simulink model "VMC_Integration"  (R2024a)
settings: Solver=FixedStepDiscrete  StartTime=0.0  StopTime=10.0  FixedStep=0.005  RelTol=1e-3
undefined symbols (not defined in the file): Degree_To_Rad_Factor
libraries: simulink x24, slpidlib x5
(part 3 of 3)

== system VMC_Integration/Traction_Control/LimitedSlipDifferential/Subsystem ==
  LSD_Enable : Inport
  Controller_Setting : Inport  Port=2
  Bus Selector : BusSelector  OutputSignals=TC_Controller.TC_PID.TC_P,TC_Controller.TC_PID.TC_I,TC_Controller.TC_PID.TC_D
  Constant15 : Constant  Value=100  OutDataTypeStr=single  SampleTime=-1
  Data Type Conversion : DataTypeConversion  OutDataTypeStr=single  SaturateOnIntegerOverflow=off  RndMeth=Floor
  Demux : Demux
  Logical Operator1 : Logic  Operator=NAND  AllPortsSameDT=off  OutDataTypeStr=boolean
  Logical Operator2 : Logic  Operator=NAND  AllPortsSameDT=off  OutDataTypeStr=boolean
  Mux5 : Mux  Inputs=5
  Terminator : Terminator
  PID_Setting : Outport
  wires:
  Demux/4 -> Logical Operator1/2
  Demux/2 -> Logical Operator2/1
  Bus Selector/2 -> Mux5/2  "<TC_I>"
  Data Type Conversion/1 -> Mux5/5
  Mux5/1 -> PID_Setting/1  "PID_ParaFL"
  Constant15/1 -> Mux5/4  "N"
  Logical Operator1/1 -> Data Type Conversion/1
  Demux/3 -> Logical Operator2/2
  Demux/1 -> Logical Operator1/1
  Bus Selector/3 -> Mux5/3  "<TC_D>"
  LSD_Enable/1 -> Demux/1
  Bus Selector/1 -> Mux5/1  "<TC_P>"
  Logical Operator2/1 -> Terminator/1
  Controller_Setting/1 -> Bus Selector/1

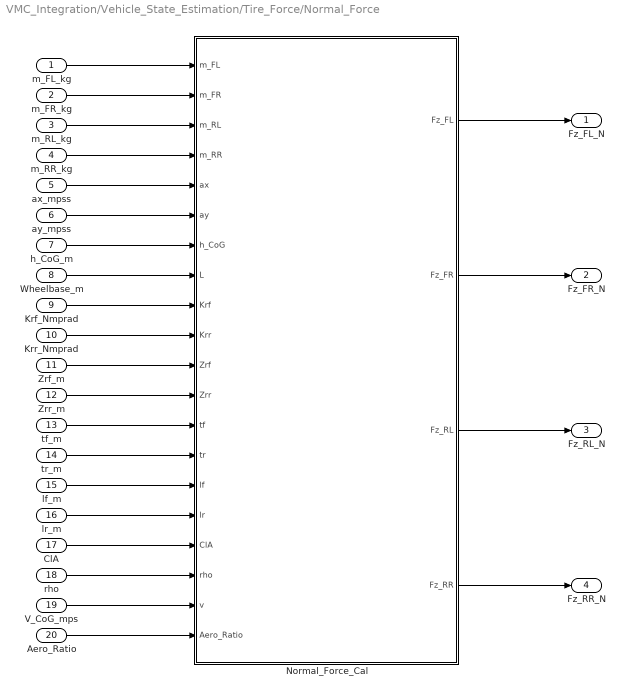
== system VMC_Integration/Vehicle_State_Estimation/Tire_Force/Normal_Force ==
  m_FL_kg : Inport
  m_FR_kg : Inport  Port=2
  m_RL_kg : Inport  Port=3
  m_RR_kg : Inport  Port=4
  ax_mpss : Inport  Port=5
  ay_mpss : Inport  Port=6
  h_CoG_m : Inport  Port=7
  Wheelbase_m : Inport  Port=8
  Krf_Nmprad : Inport  Port=9
  Krr_Nmprad : Inport  Port=10
  Zrf_m : Inport  Port=11
  Zrr_m : Inport  Port=12
  tf_m : Inport  Port=13
  tr_m : Inport  Port=14
  lf_m : Inport  Port=15
  lr_m : Inport  Port=16
  ClA : Inport  Port=17
  rho : Inport  Port=18
  V_CoG_mps : Inport  Port=19
  Aero_Ratio : Inport  Port=20
  Normal_Force_Cal : MATLAB Function  TreatAsAtomicUnit=on
  Fz_FL_N : Outport
  Fz_FR_N : Outport  Port=2
  Fz_RL_N : Outport  Port=3
  Fz_RR_N : Outport  Port=4
  wires:
  m_FL_kg/1 -> Normal_Force_Cal/1(m_FL)
  m_FR_kg/1 -> Normal_Force_Cal/2(m_FR)
  m_RL_kg/1 -> Normal_Force_Cal/3(m_RL)
  m_RR_kg/1 -> Normal_Force_Cal/4(m_RR)
  ax_mpss/1 -> Normal_Force_Cal/5(ax)
  ay_mpss/1 -> Normal_Force_Cal/6(ay)
  h_CoG_m/1 -> Normal_Force_Cal/7(h_CoG)
  Wheelbase_m/1 -> Normal_Force_Cal/8(L)
  Krf_Nmprad/1 -> Normal_Force_Cal/9(Krf)
  Krr_Nmprad/1 -> Normal_Force_Cal/10(Krr)
  Zrf_m/1 -> Normal_Force_Cal/11(Zrf)
  Zrr_m/1 -> Normal_Force_Cal/12(Zrr)
  tf_m/1 -> Normal_Force_Cal/13(tf)
  tr_m/1 -> Normal_Force_Cal/14(tr)
  lf_m/1 -> Normal_Force_Cal/15(lf)
  lr_m/1 -> Normal_Force_Cal/16(lr)
  ClA/1 -> Normal_Force_Cal/17(ClA)
  rho/1 -> Normal_Force_Cal/18(rho)
  V_CoG_mps/1 -> Normal_Force_Cal/19(v)
  Aero_Ratio/1 -> Normal_Force_Cal/20(Aero_Ratio)
  Normal_Force_Cal/1(Fz_FL) -> Fz_FL_N/1
  Normal_Force_Cal/2(Fz_FR) -> Fz_FR_N/1
  Normal_Force_Cal/3(Fz_RL) -> Fz_RL_N/1
  Normal_Force_Cal/4(Fz_RR) -> Fz_RR_N/1

== system VMC_Integration/Vehicle_State_Estimation/Tractive_Regen_Torque/REG_Enable ==
  Brake_Demand_Pct : Inport  OutDataTypeStr=single
  MotorSpeed_Array_rpm : Inport  Port=2  OutDataTypeStr=single
  REG_Button_Bool : Inport  Port=3  OutDataTypeStr=boolean
  HV_Voltage_V : Inport  Port=4  OutDataTypeStr=single
  Compare To Constant1 : simulink/Logic and Bit Operations/Compare To Constant  relop=>  const=1500  OutDataTypeStr=boolean
  Compare To Constant2 : simulink/Logic and Bit Operations/Compare To Constant  relop=>  const=0  OutDataTypeStr=boolean
  Compare To Constant3 : simulink/Logic and Bit Operations/Compare To Constant  relop=<=  const=570  OutDataTypeStr=boolean
  Demux2 : Demux
  Logical Operator : Logic  Inputs=4  AllPortsSameDT=off  OutDataTypeStr=boolean
  Min : MinMax  Inputs=2  OutDataTypeStr=int16
  Terminator : Terminator
  Terminator1 : Terminator
  REG_Enable_Bool : Outport
  wires:
  Brake_Demand_Pct/1 -> Compare To Constant2/1
  Demux2/2 -> Terminator1/1
  HV_Voltage_V/1 -> Compare To Constant3/1
  Compare To Constant1/1 -> Logical Operator/1
  Demux2/1 -> Terminator/1
  REG_Button_Bool/1 -> Logical Operator/3
  Compare To Constant3/1 -> Logical Operator/4
  MotorSpeed_Array_rpm/1 -> Demux2/1
  Demux2/3 -> Min/1
  Min/1 -> Compare To Constant1/1
  Compare To Constant2/1 -> Logical Operator/2
  Demux2/4 -> Min/2
  Logical Operator/1 -> REG_Enable_Bool/1

== system VMC_Integration/YawRate_Controller/CalMz_FB/Avg_Wheel_Angle ==
  WheelAngle_Array_rad : Inport
  Constant : Constant  Value=2  OutDataTypeStr=single
  Demux : Demux
  Divide : Product  Inputs=*/  OutDataTypeStr=single
  Sum : Sum  OutDataTypeStr=single  AccumDataTypeStr=single
  Terminator : Terminator
  Terminator1 : Terminator
  Avg_WheelAngle_rad : Outport
  wires:
  Sum/1 -> Divide/1
  Constant/1 -> Divide/2
  Divide/1 -> Avg_WheelAngle_rad/1
  Demux/1 -> Sum/1
  Demux/2 -> Sum/2
  Demux/3 -> Terminator/1
  Demux/4 -> Terminator1/1
  WheelAngle_Array_rad/1 -> Demux/1

== system VMC_Integration/YawRate_Controller/CalMz_FB/TV_Reset ==
  Avg_WheelAngle_rad : Inport
  LateralAcceleration_mpss : Inport  Port=2
  Abs1 : Abs  OutDataTypeStr=single  SaturateOnIntegerOverflow=off
  Abs2 : Abs  OutDataTypeStr=single  SaturateOnIntegerOverflow=off
  Compare To Constant : simulink/Logic and Bit Operations/Compare To Constant  relop=<=  const=0.02  OutDataTypeStr=boolean
  Compare To Constant1 : simulink/Logic and Bit Operations/Compare To Constant  relop=<=  const=3  OutDataTypeStr=boolean
  Logical Operator : Logic  AllPortsSameDT=off  OutDataTypeStr=boolean
  TV_Reset : Outport
  wires:
  LateralAcceleration_mpss/1 -> Abs1/1
  Abs1/1 -> Compare To Constant1/1
  Logical Operator/1 -> TV_Reset/1  "TV_Reset"
  Compare To Constant/1 -> Logical Operator/1  "TV_Reset1"
  Compare To Constant1/1 -> Logical Operator/2  "TV_Reset2"
  Avg_WheelAngle_rad/1 -> Abs2/1
  Abs2/1 -> Compare To Constant/1

== system VMC_Integration/YawRate_Controller/CalcMzDes_FF/Avg_Wheel_Angle ==
  WheelAngle_Array_rad : Inport
  Constant : Constant  Value=2  OutDataTypeStr=single
  Demux : Demux
  Divide : Product  Inputs=*/  OutDataTypeStr=single
  Sum : Sum  OutDataTypeStr=single  AccumDataTypeStr=single
  Terminator : Terminator
  Terminator1 : Terminator
  Avg_WheelAngle_rad : Outport
  wires:
  Sum/1 -> Divide/1
  Constant/1 -> Divide/2
  Divide/1 -> Avg_WheelAngle_rad/1
  Demux/1 -> Sum/1
  Demux/2 -> Sum/2
  Demux/3 -> Terminator/1
  Demux/4 -> Terminator1/1
  WheelAngle_Array_rad/1 -> Demux/1

== system VMC_Integration/YawRate_Controller/CalcMzDes_FF/Integrator ==
  dx : Inport  PortDimensions=[5,1]
  Demux : Demux  Outputs=5
  Mux : Mux  Inputs=5
  integrator1 : Subsystem
  integrator2 : Subsystem
  integrator3 : Subsystem
  integrator4 : Subsystem
  integrator5 : Subsystem
  x : Outport  PortDimensions=[5,1]
  wires:
  dx/1 -> Demux/1
  Demux/1 -> integrator1/1(In)
  Demux/2 -> integrator2/1(In)
  Demux/3 -> integrator3/1(In)
  Demux/4 -> integrator4/1(In)
  Demux/5 -> integrator5/1(In)
  integrator1/1(Out) -> Mux/1
  integrator2/1(Out) -> Mux/2
  integrator3/1(Out) -> Mux/3
  integrator4/1(Out) -> Mux/4
  integrator5/1(Out) -> Mux/5
  Mux/1 -> x/1

== system VMC_Integration/YawRate_Controller/CalcMzDes_FF/Integrator/integrator1 ==
  In : Inport
  Add : Sum
  Add1 : Sum
  Constant : Constant  Value=0.005  OutDataTypeStr=single
  Constant1 : Constant  Value=0  OutDataTypeStr=single
  Delay1 : Delay  DelayLength=1  InitialCondition=0
  Divide : Product  Inputs=**
  Out : Outport  VectorParamsAs1DForOutWhenUnconnected=off
  wires:
  In/1 -> Divide/1
  Constant/1 -> Divide/2
  Divide/1 -> Add/1
  Delay1/1 -> Add/2, Add1/2
  Constant1/1 -> Add1/1
  Add/1 -> Delay1/1
  Add1/1 -> Out/1

== system VMC_Integration/YawRate_Controller/CalcMzDes_FF/Integrator/integrator2 ==
  In : Inport
  Add : Sum
  Add1 : Sum
  Constant : Constant  Value=0.005  OutDataTypeStr=single
  Constant1 : Constant  Value=0  OutDataTypeStr=single
  Delay1 : Delay  DelayLength=1  InitialCondition=0
  Divide : Product  Inputs=**
  Out : Outport  VectorParamsAs1DForOutWhenUnconnected=off
  wires:
  Add1/1 -> Out/1
  Add/1 -> Delay1/1
  Constant1/1 -> Add1/1
  Delay1/1 -> Add1/2, Add/2
  Divide/1 -> Add/1
  Constant/1 -> Divide/2
  In/1 -> Divide/1

== system VMC_Integration/YawRate_Controller/CalcMzDes_FF/Integrator/integrator3 ==
  In : Inport
  Add : Sum
  Add1 : Sum
  Constant : Constant  Value=0.005  OutDataTypeStr=single
  Constant1 : Constant  Value=0  OutDataTypeStr=single
  Delay1 : Delay  DelayLength=1  InitialCondition=0
  Divide : Product  Inputs=**
  Out : Outport  VectorParamsAs1DForOutWhenUnconnected=off
  wires:
  In/1 -> Divide/1
  Constant/1 -> Divide/2
  Divide/1 -> Add/1
  Delay1/1 -> Add/2, Add1/2
  Constant1/1 -> Add1/1
  Add/1 -> Delay1/1
  Add1/1 -> Out/1

== system VMC_Integration/YawRate_Controller/CalcMzDes_FF/Integrator/integrator4 ==
  In : Inport
  Add : Sum
  Add1 : Sum
  Constant : Constant  Value=0.005  OutDataTypeStr=single
  Constant1 : Constant  Value=0  OutDataTypeStr=single
  Delay1 : Delay  DelayLength=1  InitialCondition=0
  Divide : Product  Inputs=**
  Out : Outport  VectorParamsAs1DForOutWhenUnconnected=off
  wires:
  In/1 -> Divide/1
  Constant/1 -> Divide/2
  Divide/1 -> Add/1
  Delay1/1 -> Add/2, Add1/2
  Constant1/1 -> Add1/1
  Add/1 -> Delay1/1
  Add1/1 -> Out/1

== system VMC_Integration/YawRate_Controller/CalcMzDes_FF/Integrator/integrator5 ==
  In : Inport
  Add : Sum
  Add1 : Sum
  Constant : Constant  Value=0.005  OutDataTypeStr=single
  Constant1 : Constant  Value=0  OutDataTypeStr=single
  Delay1 : Delay  DelayLength=1  InitialCondition=0
  Divide : Product  Inputs=**
  Out : Outport  VectorParamsAs1DForOutWhenUnconnected=off
  wires:
  Add1/1 -> Out/1
  Add/1 -> Delay1/1
  Constant1/1 -> Add1/1
  Delay1/1 -> Add1/2, Add/2
  Divide/1 -> Add/1
  Constant/1 -> Divide/2
  In/1 -> Divide/1

== matlab function VMC_Integration/Vehicle_State_Estimation/Vehicle_CoG_Calculation ==
  data: Overall_Mass output; CoG_From_Front output; CoG_From_Rear output; CoG_Height output; m_FL input; m_FR input; m_RL input; m_RR input; m_RL1 input; m_RR1 input; l input; h input; r input
function [Overall_Mass,CoG_From_Front,CoG_From_Rear,CoG_Height] = fcn(m_FL,m_FR,m_RL,m_RR,m_RL1,m_RR1,l,h,r) 
%%h=前桥被举升的高度，mass_RL1及mass_RL2分别为左后及右后轮被举升后的载荷(参考：测量质心高度的方法)

Overall_Mass = m_FL + m_FR + m_RL + m_RR;
CoG_From_Front = l * (m_RL + m_RR) / Overall_Mass;
CoG_From_Rear = l * (m_FL + m_FR) / Overall_Mass;
CoG_Height = l * (m_RL1 + m_RR1 - m_RL - m_RR) / (Overall_Mass * h) * sqrt(l^2 - h^2) + r;

== matlab function VMC_Integration/YawRate_Controller/CalcMzDes_FF/MATLAB Function ==
  data: Kf input; v_char output; Kr input; lr input; lf input; m input
function v_char = fcn(Kf, Kr, lr, lf, m)

v_char = single((Kf*Kr*lr^2) / (m*(Kr*lr-Kf*lf)));
end

== matlab function VMC_Integration/Power_Limitation/Power_Estimation/MATLAB Function ==
  data: Torque input; Eta input; Est_Power output; Speed input
function Est_Power  = fcn(Torque, Eta, Speed)

P = zeros(4,1);
Est_Power = 0;
for i=1:1:4
    P(i) = Torque(i)*Speed(i)*pi/30/1000/Eta(i);
    Est_Power = Est_Power + P(i);
end

== matlab function VMC_Integration/Power_Limitation/FeedForward_PowerLimit ==
  data: factor output; Torque input; Torque_out output; Est_Power input; Tractive_Limit_Power input; Regen_Limit_Power input
function [factor, Torque_out] = fcn(Torque, Est_Power, Tractive_Limit_Power, Regen_Limit_Power)

if Est_Power >= Tractive_Limit_Power
    factor = Tractive_Limit_Power / Est_Power;
    Torque_out = Torque * factor;
elseif Est_Power <= Regen_Limit_Power
    factor = Regen_Limit_Power / Est_Power;
    Torque_out = Torque * factor;
else
    factor = single(1);
    Torque_out = Torque;

end

== matlab function VMC_Integration/Power_Limitation/MATLAB Function ==
  data: Torque input; Torque_out output; Tractive_Limit_Power input; Regen_Limit_Power input; Act_Power input
function Torque_out = fcn(Torque, Tractive_Limit_Power, Regen_Limit_Power, Act_Power)

    x = [-inf, Regen_Limit_Power, Regen_Limit_Power+5, Tractive_Limit_Power-5, Tractive_Limit_Power, inf];
    y = [0, 0, 1, 1, 0, 0];
    
    scale_factor = interp1(x, y, Act_Power, 'linear', 'extrap');
    
    Torque_out = scale_factor * Torque;
end

== matlab function VMC_Integration/Vehicle_State_Estimation/Velocity_Estimation/CoG_Linear_Velocity_Calculation ==
  data: Actual_Yaw_Rate input; CoG_Vx output; OS_Vx input; OS_Vy input; OS_X_Distance input; OS_Y_Distance input; CoG_Vy output; CoG_V output; OS_V output
function [CoG_Vx, CoG_Vy, CoG_V, OS_V] = fcn(Actual_Yaw_Rate, OS_Vx, OS_Vy, OS_X_Distance ,OS_Y_Distance)
    CoG_Vx = OS_Vx / 3.6 + Actual_Yaw_Rate * OS_Y_Distance;
    CoG_Vy = OS_Vy / 3.6 - Actual_Yaw_Rate * OS_X_Distance;
    CoG_V = single(sqrt(CoG_Vx ^ 2 + CoG_Vy ^ 2));
    OS_V = single(sqrt((OS_Vx / 3.6) ^ 2 + (OS_Vy / 3.6) ^ 2));
end

== matlab function VMC_Integration/YawRate_Controller/CalcMzDes_FF/FF_Yaw_Moment_Calc ==
  data: x input; dx output; delta_s input; v_x input; faktor_GV_stat input; faktor_T_psi input; faktor_omega_e input; faktor_D input; dpsi_des output; Mz_add_FF output; l_R input; l_F input; m input; I_zz input; C_alphaF input; C_alphaR input; i_L input; v_char input; v_thr_act input; Control_active_flag output
function [dx, dpsi_des, Mz_add_FF, Control_active_flag] = ...
    FF_Yaw_Moment_Calc(x, delta_s, v_x, faktor_GV_stat, faktor_T_psi, faktor_omega_e, faktor_D, l_R, l_F, m, I_zz, C_alphaF, C_alphaR, i_L, v_char, v_thr_act)
%% Header
% Function for calculating the refernce yaw rate and the feed foward yaw
% moment

% Written by Markus Ortner / AVL CDTE H_C / Dez 2018

% Inputs
% - x:                controler state vector
% - delta_s           steering wheel angle
% - v_x               vehicle velocity
% - faktor_GV_stat    factor for scaling the steady state yaw gain 
% - faktor_T_psi      factor for scaling the yaw response time 
% - faktor_omega_e    factor for scaling the undamped eigenfrequency
% - faktor_D          factor for scaling the damping coefficient 
% - l_R               distance center of gravity to the front axle 
% - l_F               distance center of gravity to the rear axle 
% - m                 vehicles mass 
% - I_zz              vehilces inertia around the certical axle 
% - C_alphaF          front axle side slip stiffness 
% - C_alphaR          rear axle side slip stiffness 
% - i_L               steering velocity 
% - v_char            characteristic velocity 
% - v_thr_act         velocity threshold, above this threshold controller is active, has to be bigger than 0

% Outputs
% - dx:                   controller state derivative vector
% - dpsi_des              refernce yaw rate
% - Mz_add_FF             feed forward yaw moment
% - Control_active_flag   flag variable if controller is active

%% split state vektor
x_ref = x(1:2);
x_FF = x(3:5);

%% Recalculated parameter

% calculated wheelbase
l = l_F+l_R;

%% parameter calcutlatation for desired yaw transfer function

% Transfer function G_deltas_dpsi = GV_stat0 * (1+Tpsi*s) / (1+(2*D/omega_e)+(1/omega_e^2)s^2)

% parameter of the baselines vehicle of the linear two wheel model
G_deltas_dpsi_stat0     = v_x/(l*(1+v_x^2/v_char^2));
Tpsi0                   = (m*v_x*l_F)/(C_alphaR*l);
omegae0                 = sqrt((C_alphaF*C_alphaR*l^2+m*v_x^2*(C_alphaR*l_R-C_alphaF*l_F))/(I_zz*m*(v_x+eps)^2));
D_0                     = (m*(C_alphaF*l_F^2+C_alphaR*l_R^2)+I_zz*(C_alphaF+C_alphaR))/(2*I_zz*m*(v_x+eps))/omegae0;

%  parameters of the desiered yaw transfer function 
G_deltas_dpsi_des_stat  = G_deltas_dpsi_stat0*faktor_GV_stat;
T_psi                   = Tpsi0*faktor_T_psi;
omega_e                 = omegae0*faktor_omega_e;
D                       = D_0*faktor_D;

%% Transfer handwheel angel to road wheel angle
delta_F = delta_s/i_L;

%% Rearenge yaw transfer function to state space format
a_0_ref = omega_e^2;
a_1_ref = 2*D*omega_e;
b_0_ref = G_deltas_dpsi_des_stat*omega_e^2;
b_1_ref = G_deltas_dpsi_des_stat*T_psi*omega_e^2;

A_ref = [0,1;-a_0_ref, -a_1_ref];
b_ref = [0;1];

c_ref = [b_0_ref, b_1_ref];
d_ref = 0;

dx_ref = A_ref*x_ref+b_ref*delta_F;
dpsi_des_LRM = c_ref*x_ref+d_ref*delta_F;


%% Rearenge Feed forward yaw moment transfer function to state space format
    % coefficient calculated in seperate MATLAB skrip using MATLAB's
    % symbolic toolbox
    
b_0_FF = (C_alphaF*C_alphaR*G_deltas_dpsi_des_stat*l_F^2*omega_e^2 + ...
    2*C_alphaF*C_alphaR*G_deltas_dpsi_des_stat*l_F*l_R*omega_e^2 - ...
    C_alphaF*G_deltas_dpsi_des_stat*m*l_F*omega_e^2*v_x^2 - C_alphaF*C_alphaR*l_F*omega_e^2*v_x + ...
    C_alphaF*C_alphaR*G_deltas_dpsi_des_stat*l_R^2*omega_e^2 + C_alphaR*G_deltas_dpsi_des_stat*m*l_R*omega_e^2*v_x^2 - ...
    C_alphaF*C_alphaR*l_R*omega_e^2*v_x)/(m*v_x^2);
b_1_FF = (C_alphaF*G_deltas_dpsi_des_stat*I_zz*omega_e^2*v_x - C_alphaF*l_F*m*omega_e^2*v_x^2 + ...
    C_alphaR*G_deltas_dpsi_des_stat*I_zz*omega_e^2*v_x + C_alphaF*C_alphaR*G_deltas_dpsi_des_stat*T_psi*l_F^2*omega_e^2 + ...
    C_alphaF*C_alphaR*G_deltas_dpsi_des_stat*T_psi*l_R^2*omega_e^2 + C_alphaF*G_deltas_dpsi_des_stat*l_F^2*m*omega_e^2*v_x + ...
    C_alphaR*G_deltas_dpsi_des_stat*l_R^2*m*omega_e^2*v_x - 2*C_alphaF*C_alphaR*D*l_F*omega_e*v_x - ...
    2*C_alphaF*C_alphaR*D*l_R*omega_e*v_x + 2*C_alphaF*C_alphaR*G_deltas_dpsi_des_stat*T_psi*l_F*l_R*omega_e^2 - ...
    C_alphaF*G_deltas_dpsi_des_stat*T_psi*l_F*m*omega_e^2*v_x^2 + ...
    C_alphaR*G_deltas_dpsi_des_stat*T_psi*l_R*m*omega_e^2*v_x^2)/(m*v_x^2);
b_2_FF = (G_deltas_dpsi_des_stat*I_zz*m*omega_e^2*v_x^2 - C_alphaF*C_alphaR*l_R*v_x - ...
    C_alphaF*C_alphaR*l_F*v_x - 2*C_alphaF*D*l_F*m*omega_e*v_x^2 + ...
    C_alphaF*G_deltas_dpsi_des_stat*I_zz*T_psi*omega_e^2*v_x + ...
    C_alphaR*G_deltas_dpsi_des_stat*I_zz*T_psi*omega_e^2*v_x + ...
    C_alphaF*G_deltas_dpsi_des_stat*T_psi*l_F^2*m*omega_e^2*v_x + ...
    C_alphaR*G_deltas_dpsi_des_stat*T_psi*l_R^2*m*omega_e^2*v_x)/(m*v_x^2);
b_3_FF =  -(- G_deltas_dpsi_des_stat*I_zz*T_psi*m*omega_e^2*v_x^2 + C_alphaF*l_F*m*v_x^2)/(m*v_x^2);
a_0_FF = (omega_e^2*(C_alphaF + C_alphaR))/(m*v_x);
a_1_FF = (m*omega_e^2*v_x^2 + 2*D*(C_alphaF + C_alphaR)*omega_e*v_x)/(m*v_x^2);
a_2_FF = (2*D*m*omega_e*v_x^2 + (C_alphaF + C_alphaR)*v_x)/(m*v_x^2);

A_FF = [0, 1, 0; 0, 0, 1; -a_0_FF, -a_1_FF, -a_2_FF];
b_FF = [0;0;1];

c_FF = [b_0_FF-b_3_FF*a_0_FF, b_1_FF-b_3_FF*a_1_FF,  b_2_FF-b_3_FF*a_2_FF];
d_FF = b_3_FF;

dx_FF = A_FF*x_FF+b_FF*delta_F;
Mz_add_FF_LRM = c_FF*x_FF+d_FF*delta_F;

%% Assign Outputs and decide if contoller is active or not

dx = single(zeros(5,1));
Mz_add_FF = single(0);
dpsi_des = single(0);
Control_active_flag = false;

if v_x>=v_thr_act
    dx = [dx_ref;dx_FF];
    Mz_add_FF = Mz_add_FF_LRM;
    dpsi_des =  dpsi_des_LRM;
    Control_active_flag = true;
end

== matlab function VMC_Integration/Vehicle_State_Estimation/Wheel_State/WhlSpdActlCal ==
  data: WhlSpdActlFL output; Gear_Ratio input; MotSpdByrpm input; WhlSpdActlFR output; WhlSpdActlRL output; WhlSpdActlRR output
function [WhlSpdActlFL, WhlSpdActlFR, WhlSpdActlRL, WhlSpdActlRR] = fcn(Gear_Ratio, MotSpdByrpm)
WhlSpdActlFL = single(MotSpdByrpm(1) * 2 * pi / Gear_Ratio / 60);
WhlSpdActlFR = single(MotSpdByrpm(2) * 2 * pi / Gear_Ratio / 60);
WhlSpdActlRL = single(MotSpdByrpm(3) * 2 * pi / Gear_Ratio / 60);
WhlSpdActlRR = single(MotSpdByrpm(4) * 2 * pi / Gear_Ratio / 60);
end

== matlab function VMC_Integration/Torque_Allocation/Subsystem2/mu_x_FL ==
  data: mu input; mu_x output; mu_y input
function mu_x = fcn(mu, mu_y)

if mu^2 - mu_y^2 > 0
    mu_x = single(sqrt(mu^2 - mu_y^2));
else
    mu_x = single(0.01);
end

== matlab function VMC_Integration/Torque_Allocation/Subsystem2/mu_x_FR ==
  data: mu input; mu_x output; mu_y input
function mu_x = fcn(mu, mu_y)

if mu^2 - mu_y^2 > 0
    mu_x = single(sqrt(mu^2 - mu_y^2));
else
    mu_x = single(0.01);
end

== matlab function VMC_Integration/Torque_Allocation/Subsystem2/mu_x_RL ==
  data: mu input; mu_x output; mu_y input
function mu_x = fcn(mu, mu_y)

if mu^2 - mu_y^2 > 0
    mu_x = single(sqrt(mu^2 - mu_y^2));
else
    mu_x = single(0.01);
end

== matlab function VMC_Integration/Torque_Allocation/Subsystem2/mu_x_RR ==
  data: mu input; mu_x output; mu_y input
function mu_x = fcn(mu, mu_y)

if mu^2 - mu_y^2 > 0
    mu_x = single(sqrt(mu^2 - mu_y^2));
else
    mu_x = single(0.01);
end

== matlab function VMC_Integration/Torque_Allocation/Torque_Distribution ==
  data: T_tot input; T output single; M_ref input; lf input; bf input; br input; theta_FL input; theta_FR input; i input; r0 input; Fz input; mu input; Max_Motor_Torque input; Max_Req_Torque input; Req_Demand input; exitflag output; ActExtYaw output; iA_p input; iA output
function [T, exitflag,ActExtYaw, iA]   = fcn(T_tot, M_ref, lf, bf, br, theta_FL, theta_FR, i, r0, Fz, mu, Max_Motor_Torque, Max_Req_Torque, Req_Demand, iA_p)
% Define Input from outside
% CoG from Front
% Front Axle Width
% Rear Axle Width
% Gear Ratio
% Rolling Radius

if Req_Demand == 0
    t_max = single(Max_Motor_Torque);
    t_min = single(Max_Req_Torque);
else
    t_max = single([0;0;0;0]);
    t_min = single(Max_Req_Torque);
end
% Undefined Factor

k1 = single(10); 
k2=single(0.01); k3=single(1);

% if Req_Demand == 0
%     T_f = T_tot * 0.3;
%     T_r = T_tot * 0.7;
% else
%     T_f = T_tot * 0.7;
%     T_r = T_tot * 0.3;
% end

% Preparation
% G1
h_FL = single((lf*sin(theta_FL) - bf*cos(theta_FL)/2) * i / r0);
h_FR = single((lf*sin(theta_FR) + bf*cos(theta_FR)/2) * i / r0);
h_RL = single(-(br / 2) * (i / r0));
h_RR = single((br / 2) * (i / r0));
H = single([h_FL h_FR h_RL h_RR]);
G1 = single(2*[
    h_FL^2, h_FL*h_FR, h_FL*h_RL, h_FL*h_RR;
    h_FR*h_FL, h_FR^2, h_FR*h_RL, h_FR*h_RR;
    h_RL*h_FL, h_RL*h_FR, h_RL^2, h_RL*h_RR;
    h_RR*h_FL, h_RR*h_FR, h_RR*h_RL, h_RR^2
]);

% G2
t_sat = single(zeros(4,1));
t_sat(1) =  single(Fz(1) * mu(1) * r0 / i);
t_sat(2) =  single(Fz(2) * mu(2) * r0 / i);
t_sat(3) =  single(Fz(3) * mu(3) * r0 / i);
t_sat(4) =  single(Fz(4) * mu(4) * r0 / i);

for i=1:4
    if t_sat(i) == 0
        t_sat(i) = 0.01;
    end
end

G2 = single([
    (1/(t_sat(1)))^2, 0, 0, 0;
    0, (1/(t_sat(2)))^2, 0, 0;
    0, 0, (1/(t_sat(3)))^2, 0;
    0, 0, 0, (1/(t_sat(4)))^2
]);

G3 = single([
    1, 0, 0, 0;
    0, 1, 0, 0;
    0, 0, 1, 0;
    0, 0, 0, 1
]);

G = zeros(4,4);
G = single(k1*G1 + k2*G2 + k3*G3);
f = single(zeros(4,1));
f = single(k1 * (-2 * M_ref * H'));

if Req_Demand == 0
    T_sat = min(t_max(1), t_sat(1)) + min(t_max(2), t_sat(2)) + min(t_max(3), t_sat(3)) + min(t_max(4), t_sat(4));
    if T_tot > T_sat
        T_tot  = T_sat;
    end
else
    T_sat1 = max(t_min(1), -t_sat(1)) + max(t_min(2), -t_sat(2)) + max(t_min(3), -t_sat(3)) + max(t_min(4), -t_sat(4));
    T_sat2 = sum(Max_Req_Torque);
    T_tot = max([T_tot, T_sat1, T_sat2]);
end

% Boundary Conditions
A_eq = single([1 1 1 1]);
b_eq = single(T_tot);

% A_eq = single([1 1 0 0; 0 0 1 1]);
% b_eq = single([T_f; T_r]);


A_ineq = single([
    1, 0, 0, 0;
    0, 1, 0, 0;
    0, 0, 1, 0;
    0, 0, 0, 1;
    -1, 0, 0, 0;
    0, -1, 0, 0;
    0, 0, -1, 0;
    0, 0, 0, -1
]);
if Req_Demand == 0
    b_ineq = single([
        min(t_max(1), t_sat(1));
        min(t_max(2), t_sat(2));
        min(t_max(3), t_sat(3));
        min(t_max(4), t_sat(4));
        -max(t_min(1), -t_sat(1));
        -max(t_min(2), -t_sat(2));
        -max(t_min(3), -t_sat(3));
        -max(t_min(4), -t_sat(4))
    ]);
else
    b_ineq = single([
        0;
        0;
        0;
        0;
        -max(t_min(1), -t_sat(1));
        -max(t_min(2), -t_sat(2));
        -max(t_min(3), -t_sat(3));
        -max(t_min(4), -t_sat(4))
    ]);
end
% Solve

% options = mpcInteriorPointOptions('single');
% options.MaxIterations = single(50);
% options.ConstraintTolerance = single(1e-2);
% options.OptimalityTolerance = single(1e-2);
% options.ComplementarityTolerance = single(1e-4);
% options.StepTolerance = single(1e-4);
% [T_QP, exitflag] = mpcInteriorPointSolver(G,f,A_ineq,b_ineq,A_eq,b_eq,single([0;0;0;0]),options);

options = mpcActiveSetOptions('single');
options.MaxIterations = single(100);
options.ConstraintTolerance = single(1e-3);

% T_QP = single(zeros(4,1));
[T_QP, exitflag, iA] = mpcActiveSetSolver(G,f,A_ineq,b_ineq,A_eq,b_eq,iA_p,options);

T = single([0;0;0;0]);
Tot_Fz = Fz(1) + Fz(2) + Fz(3) + Fz(4);
if exitflag <= 0
    T(1) = T_tot * Fz(1) / Tot_Fz;
    T(2) = T_tot * Fz(2) / Tot_Fz;
    T(3) = T_tot * Fz(3) / Tot_Fz;
    T(4) = T_tot * Fz(4) / Tot_Fz;
else
    T = T_QP;
end

% Output_Torque
% if Req_Demand == 0
%     T_sat = min(t_max(1), t_sat(1)) + min(t_max(2), t_sat(2)) + min(t_max(3), t_sat(3)) + min(t_max(4), t_sat(4));
%     if exitflag <= 0
%         if T_sat < T_tot
%             T_tot = T_sat;
%         end 
%         T = [
%             min([T_tot * Fz(1) / sum(Fz),t_max(1),t_sat(1)]);
%             min([T_tot * Fz(2) / sum(Fz),t_max(2),t_sat(2)]);
%             min([T_tot * Fz(3) / sum(Fz),t_max(3),t_sat(3)]);
%             min([T_tot * Fz(4) / sum(Fz),t_max(4),t_sat(4)]);
%             ];
%     else
%         T = T_temp;
%     end
% else
%     T_sat = max(t_min(1), -t_sat(1)) + max(t_min(2), -t_sat(2)) + max(t_min(3), -t_sat(3)) + max(t_min(4), -t_sat(4));
%     if exitflag <= 0
%         if T_sat < T_tot
%             T_tot = T_sat;
%         end 
%         T = [
%             max([T_tot * Fz(1) / sum(Fz),t_min(1),-t_sat(1)]);
%             max([T_tot * Fz(2) / sum(Fz),t_min(2),-t_sat(2)]);
%             max([T_tot * Fz(3) / sum(Fz),t_min(3),-t_sat(3)]);
%             max([T_tot * Fz(4) / sum(Fz),t_min(4),-t_sat(4)]);
%             ];
%     else
%         T = T_temp;
%     end
% end
ActExtYaw = H*T;
end

== matlab function VMC_Integration/Vehicle_State_Estimation/Wheel_State/WhlSpdRefsCal ==
  data: WhlSpdRefFL output; CoG_vx input; CoG_vy input; WhlSpdRefFR output; WhlSpdRefRL output; WhlSpdRefRR output; Yawrate input; WheelAngle input; lf input; lr input; tf input; tr input; Offset_CoG_y input
function [WhlSpdRefFL, WhlSpdRefFR, WhlSpdRefRL, WhlSpdRefRR] = fcn(CoG_vx,CoG_vy, Yawrate, WheelAngle, lf, lr, tf, tr, Offset_CoG_y)

% Created by Yichao Zhu on 12/03/2025
% Detailed calculations on Feishu

% Inputs:
    % CoG_vx (single): Longitudinal speed at center of gravity
    % CoG_vy (single): Lateral speed at center of gravity
    % Yawrate (single): Vehicle yaw rate
    % WheelAngle ([4x1] single): Four wheel angles
    % lf (single): Distance from CoG to the front axle
    % lr (single): Distance from CoG to the rear axle
    % tf ([2x1] single): Wheelbase of front axle
    % tr ([2x1] single): Wheelbase of rear axle
    % Offset_CoG_y (single): Offset of CoG to vehicle's X axle

% Outputs
    % WhlSpdRef ([2x1] single): Wheel longitudinal and lateral speeds

FL_Matrix = [
    cos(WheelAngle(1)), sin(WheelAngle(1));
    -sin(WheelAngle(1)), cos(WheelAngle(1))
    ] * [
    1, 0, -(tf(1)-Offset_CoG_y);
    0, 1, lf
    ];

FR_Matrix = [
    cos(WheelAngle(2)), sin(WheelAngle(2));
    -sin(WheelAngle(2)), cos(WheelAngle(2))
    ] * [
    1, 0, (tf(2)+Offset_CoG_y);
    0, 1, lf
    ];

RL_Matrix = [
    cos(WheelAngle(3)), sin(WheelAngle(3));
    -sin(WheelAngle(3)), cos(WheelAngle(3))
    ] * [
    1, 0, -(tr(1)-Offset_CoG_y);
    0, 1, -lr
    ];

RR_Matrix = [
    cos(WheelAngle(4)), sin(WheelAngle(4));
    -sin(WheelAngle(4)), cos(WheelAngle(4))
    ] * [
    1, 0, (tr(2)+Offset_CoG_y);
    0, 1, -lr
    ];

state_vector = [
    CoG_vx;
    CoG_vy;
    Yawrate
    ];

% WhlSpdRef = [vx_ref; vy_ref]
WhlSpdRefFL = FL_Matrix * state_vector;
WhlSpdRefFR = FR_Matrix * state_vector;
WhlSpdRefRL = RL_Matrix * state_vector;
WhlSpdRefRR = RR_Matrix * state_vector;
end

== matlab function VMC_Integration/Vehicle_State_Estimation/Wheel_State/WhlSpdLongCal ==
  data: WhlSpdRefFL_Long output; WhlSpdRefFL input; WhlSpdRefFR input; WhlSpdRefFR_Long output; WhlSpdRefRL_Long output; WhlSpdRefRR_Long output; WhlSpdRefRL input; WhlSpdRefRR input; rolling_radius input; SA_FL output; SA_FR output; SA_RL output; SA_RR output
function [WhlSpdRefFL_Long, WhlSpdRefFR_Long, WhlSpdRefRL_Long, WhlSpdRefRR_Long, SA_FL, SA_FR, SA_RL, SA_RR] = fcn(WhlSpdRefFL, WhlSpdRefFR, WhlSpdRefRL, WhlSpdRefRR, rolling_radius)

WhlSpdRefFL_Long = WhlSpdRefFL(1)/rolling_radius;
WhlSpdRefFR_Long = WhlSpdRefFR(1)/rolling_radius;
WhlSpdRefRL_Long = WhlSpdRefRL(1)/rolling_radius;
WhlSpdRefRR_Long = WhlSpdRefRR(1)/rolling_radius;

if WhlSpdRefFL(1) < 2
    WhlSpdRefFL(1) = 2;
end
if WhlSpdRefFR(1) < 2
    WhlSpdRefFR(1) = 2;
end
if WhlSpdRefRL(1) < 2
    WhlSpdRefRL(1) = 2;
end
if WhlSpdRefRR(1) < 2
    WhlSpdRefRR(1) = 2;
end

SA_FL = atan(WhlSpdRefFL(2)/WhlSpdRefFL(1));
SA_FR = atan(WhlSpdRefFR(2)/WhlSpdRefFR(1));
SA_RL = atan(WhlSpdRefRL(2)/WhlSpdRefRL(1));
SA_RR = atan(WhlSpdRefRR(2)/WhlSpdRefRR(1));

end

== matlab function VMC_Integration/Vehicle_State_Estimation/Wheel_State/SlipRatioCal ==
  data: Actl input; SlipRate output; Ref input
function SlipRate = fcn(Actl,Ref)
    SlipRate = zeros(4,1);

    if(Actl(1) < 5)
        SlipRate(1) = single(0);
    else
        SlipRate(1) = (Actl(1)-Ref(1)) / max(Actl(1), Ref(1));
    end

    if(Actl(2) < 5)
        SlipRate(2) = single(0);
    else
        SlipRate(2) = (Actl(2)-Ref(2)) / max(Actl(2), Ref(2));
    end

    if(Actl(3) < 5)
        SlipRate(3) = single(0);
    else
        SlipRate(3) = (Actl(3)-Ref(3)) / max(Actl(3), Ref(3));
    end

    if(Actl(4) < 5)
        SlipRate(4) = single(0);
    else
        SlipRate(4) = (Actl(4)-Ref(4)) / max(Actl(4), Ref(4));
    end
end

== matlab function VMC_Integration/Vehicle_State_Estimation/Tire_Force/Normal_Force/Normal_Force_Cal ==
  data: Fz_FL output; m_FL input; m_FR input; m_RL input; m_RR input; ax input; ay input; h_CoG input; L input; Krf input; Krr input; Zrf input; Zrr input; tf input; tr input; lf input; lr input; ClA input; rho input; v input; Aero_Ratio input; Fz_FR output; Fz_RL output; Fz_RR output
function [Fz_FL, Fz_FR, Fz_RL, Fz_RR] = fcn(m_FL, m_FR, m_RL, m_RR, ax, ay, h_CoG, L, Krf, Krr, Zrf, Zrr, tf, tr, lf, lr, ClA, rho, v, Aero_Ratio)

g = 9.81;

% Static Load
Fz_FL = m_FL*g;
Fz_FR = m_FR*g;
Fz_RL = m_RL*g;
Fz_RR = m_RR*g;

% Longitudinal Load Transfer
Fz_FL = Fz_FL - m_FL*g*h_CoG*ax / (2*L);
Fz_FR = Fz_FR - m_FR*g*h_CoG*ax / (2*L);
Fz_RL = Fz_RL + m_RL*g*h_CoG*ax / (2*L);
Fz_RR = Fz_RR + m_RR*g*h_CoG*ax / (2*L);

% Lateral Load Transfer
Fz_FL = Fz_FL - m_FL*g*ay/tf*(Krf*h_CoG/(Krf+Krr) + lf*Zrf/L);
Fz_FR = Fz_FR + m_FR*g*ay/tf*(Krf*h_CoG/(Krf+Krr) + lf*Zrf/L);
Fz_RL = Fz_RL - m_RL*g*ay/tr*(Krr*h_CoG/(Krf+Krr) + lr*Zrr/L);
Fz_RR = Fz_RR + m_RR*g*ay/tr*(Krr*h_CoG/(Krf+Krr) + lr*Zrr/L);

% Aerodynamic Load
Fz_FL = Fz_FL + 0.5*rho*ClA* v^2 * Aero_Ratio *0.5;
Fz_FR = Fz_FR + 0.5*rho*ClA* v^2 * Aero_Ratio *0.5;
Fz_RL = Fz_RL + 0.5*rho*ClA* v^2 * (1-Aero_Ratio) *0.5;
Fz_RR = Fz_RR + 0.5*rho*ClA* v^2 * (1-Aero_Ratio) *0.5;

end
